simulink model "LongControlv7"  (R2019b)
settings: Solver=FixedStepAuto  StartTime=0.0  StopTime=10  FixedStep=0.01  RelTol=1e-3
InitFcn:
  | %Kp = 0.13864605;
  | %KI=0.647960817;
  | KI = 0.63153462;
  | Kp = 0.13129939;
  | M = 2.25;
  | r= 0.0425;
  | zeta = 0.08;
  | %Kp=0.1
  | Kt = 0.1292;
  | Ra = 2.7272;
  | N = 34;
  | I = 0.000016305;
  | c = 0.00006166;
  | Kb = 0.0101;
  | z=KI/Kp;
settings Model: Creator=tumu  LastModifiedBy=tumu

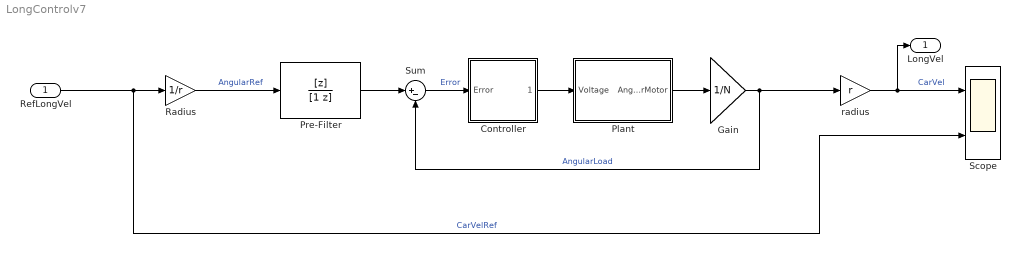
== system LongControlv7 ==
  RefLongVel : Inport
  Controller : Subsystem
  Gain : Gain  Gain=1/N
  Plant : Subsystem
  Pre-Filter : TransferFcn  Numerator=[z]  Denominator=[1 z]
  Radius : Gain  Gain=1/r
  Scope : Scope  NumInputPorts=2
  Sum : Sum  Inputs=|+-
  radius : Gain  Gain=r
  LongVel : Outport
  wires:
  Radius/1 -> Pre-Filter/1  "AngularRef"
  Pre-Filter/1 -> Sum/1
  RefLongVel/1 -> Scope/2, Radius/1  "CarVelRef"
  radius/1 -> LongVel/1, Scope/1  "CarVel"
  Gain/1 -> Sum/2, radius/1  "AngularLoad"
  Sum/1 -> Controller/1(Error)  "Error"
  Controller/1(Voltage) -> Plant/1(Voltage)
  Plant/1(AngularMotor) -> Gain/1

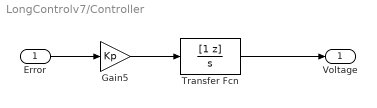
== system LongControlv7/Controller ==
  Error : Inport
  Gain5 : Gain  Gain=Kp
  Transfer Fcn : TransferFcn  Numerator=[1 z]  Denominator=[1 0]
  Voltage : Outport
  wires:
  Gain5/1 -> Transfer Fcn/1
  Error/1 -> Gain5/1
  Transfer Fcn/1 -> Voltage/1

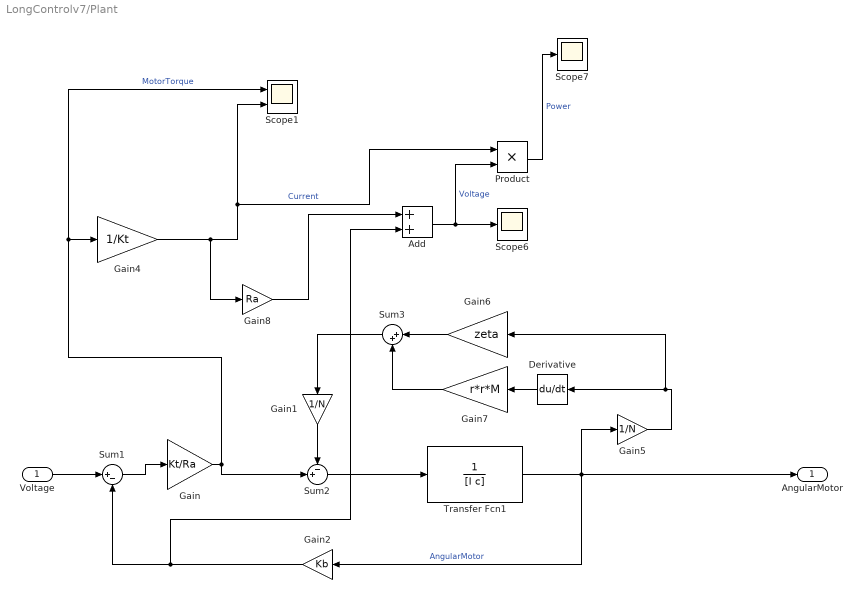
== system LongControlv7/Plant ==
  Voltage : Inport
  Add : Sum
  Derivative : Derivative
  Gain : Gain  Gain=Kt/Ra
  Gain1 : Gain  Gain=1/N
  Gain2 : Gain  Gain=Kb
  Gain4 : Gain  Gain=1/Kt
  Gain5 : Gain  Gain=1/N
  Gain6 : Gain  Gain=zeta
  Gain7 : Gain  Gain=r*r*M
  Gain8 : Gain  Gain=Ra
  Product : Product
  Scope1 : Scope  NumInputPorts=2
  Scope6 : Scope
  Scope7 : Scope
  Sum1 : Sum  Inputs=|+-
  Sum2 : Sum  Inputs=-+|
  Sum3 : Sum  Inputs=|++
  Transfer Fcn1 : TransferFcn  Denominator=[I c]
  AngularMotor : Outport
  wires:
  Gain8/1 -> Add/1
  Gain6/1 -> Sum3/1
  Gain1/1 -> Sum2/1
  Sum1/1 -> Gain/1
  Gain7/1 -> Sum3/2
  Transfer Fcn1/1 -> Gain5/1, AngularMotor/1, Gain2/1  "AngularMotor"
  Gain2/1 -> Sum1/2, Add/2
  Gain4/1 -> Scope1/2, Product/1, Gain8/1  "Current"
  Add/1 -> Product/2, Scope6/1  "Voltage"
  Sum3/1 -> Gain1/1
  Gain/1 -> Sum2/2, Scope1/1, Gain4/1  "MotorTorque"
  Derivative/1 -> Gain7/1
  Voltage/1 -> Sum1/1
  Product/1 -> Scope7/1  "Power"
  Sum2/1 -> Transfer Fcn1/1
  Gain5/1 -> Gain6/1, Derivative/1
